simulink model "FullCardioLablModel"  (R2023b)
settings: Solver=FixedStepDiscrete  StartTime=0.0  StopTime=param_sim_time  FixedStep=1/fs  MaxStep=1/fs  RelTol=1e-3
undefined symbols (not defined in the file): analyses, fdesignblkfcn, fs, gcbh, param_tot_samples
libraries: dspstat3 x13, SCGAnalysis_SignalGenerationLib x2
(part 20 of 20)

== matlab function FullCardioLablModel/SCG Analysis/Enabled SCG Analysis Subsystem/All Signals Signal Metric Characterization/SCG Systolic 3DMinS1p2pProjection Signal Metric Characterization/Spectral Distribution Calculator/Spectral Distribution Calculator ==
  data: fs input size=[1]; r_pos input; scg_signal input; entire_cycle_nsd output size=[3 1]; entire_cycle_flag input size=[1]; s1_flag input size=[1]; s2_flag input size=[1]; f_band_lo input size=[1 2]; f_band_mid input size=[1 2]; f_band_hi input size=[1 2]; s1_nsd output size=[3 1]; s2_nsd output size=[3 1]
function [entire_cycle_nsd, s1_nsd, s2_nsd] = slk_normalized_spectral_distribution_calculator(fs, r_pos,scg_signal, entire_cycle_flag, s1_flag, s2_flag, f_band_lo, f_band_mid, f_band_hi)
% Simulink function to calculate the normalized spectral distribution of the power spectral densities of the entire cyle, the s1 complex, and the s2 complex, of an input SCG signal.

% INPUTS:
% fs = sampling frequency of scg_signal.
% r_pos = index positions of the R peaks of the ecg.
% scg_signal = signal to calculate its average cycle.
% entire_cycle_flag = flag to indicate the calculation of the entire cycle spectral distribution.
% s1_flag = flag to indicate the calculation of the S1 complex spectral distribution.
% s2_flag = flag to indicate the calculation of the S2 complex spectral distribution.

% OUTPUT:
% entire_cycle_nsd = normalized spectral distribution of the entire cycle (given as 3 elements corresponding to the spectral distribution in each of the 3 bins).
% s1_nsd = normalized spectral distribution of the s1 complex (given as 3 elements corresponding to the spectral distribution in each of the 3 bins).
% s2_nsd = normalized spectral distribution of the s2 complex (given as 3 elements corresponding to the spectral distribution in each of the 3 bins).

% This function consists of three parts:
% Part 1 - Calculation of the entire cycle normalized spectral distribution.
% Part 2 - Calculation of the S1 complex normalized spectral distribution.
% Part 3 - Calculation of the S2 complex normalized spectral distribution.

coder.extrinsic('legend');
coder.extrinsic('vline');

num_cycles = length(r_pos);

pad_size = 10*fs; % The length of the zero-padded vector used to obtain sufficient frequency resolution for the FFT.

PSDs = figure;
xlabel('Frequency (Hz)')
ylabel('Power Spectral Density (mg^2)')
xlim([0 f_band_hi(2)])
title('Power Spectral Densities')
hold on

freq_axis = fs*(0:pad_size/2)/pad_size; % Frequency axis for the FFT.

%% Part 1 - Calculation of the entire cycle normalized spectral distribution.


% if entire_cycle_flag
%     
%     current_cycle_padded = zeros(pad_size,1); % Pre-initializing for speed.
%     fft_entire_cycle_mag_2_sided = zeros(pad_size,1);
%     fft_entire_cycle_mag_1_sided = zeros(pad_size/2+1,num_cycles - 1);
%     
%     for i = 1:num_cycles - 1 % The last cycle isnt considered because it's not complete.
%         
%         current_cycle = scg_signal(r_pos(i):r_pos(i+1));
%         current_cycle_length = length(current_cycle); % In samples.
%         
%         % Ensuring the current cycle has an even number of samples - necessary for FFT calculation.
%         if mod(current_cycle_length,2) > 0
%             current_cycle_length = current_cycle_length - 1;
%             current_cycle(end) = [];
%         end
%                
%         current_cycle_padded = [current_cycle; zeros(pad_size - current_cycle_length,1)];
%         fft_entire_cycle = fft(current_cycle_padded); % (Complex) FFT values.
%         fft_entire_cycle_mag_2_sided = abs(fft_entire_cycle); % Two-sided Magnitude.
%         fft_entire_cycle_mag_1_sided(:,i) = fft_entire_cycle_mag_2_sided(1:length(current_cycle_padded)/2+1); % One-sided Magnitude.
%         fft_entire_cycle_mag_1_sided(2:end-1,i) = 2*fft_entire_cycle_mag_1_sided(2:end-1,i); % Multiplying by 2 to get total power (negative + positive frequencies).
%     end
%     
%     average_entire_cycle_fft = mean(fft_entire_cycle_mag_1_sided'); % The mean magnitude FFT spectrum.
%     
%     average_entire_cycle_psd = average_entire_cycle_fft.^2; % The power spectral density - the square of the magnitude spectrum.
%     
%     % Plotting.
%     figure(PSDs); hold on;
%     plot(freq_axis,average_entire_cycle_psd)
%     
%     % Integrating along the bands to get the bandpower.
%     entire_cycle_lo_power = trapz(ceil(f_band_lo(1)/freq_axis(2)):ceil(f_band_lo(2)/freq_axis(2)),average_entire_cycle_psd(ceil(f_band_lo(1)/freq_axis(2)):ceil(f_band_lo(2)/freq_axis(2))));
%     entire_cycle_mid_power = trapz(ceil(f_band_mid(1)/freq_axis(2)):ceil(f_band_mid(2)/freq_axis(2)),average_entire_cycle_psd(ceil(f_band_mid(1)/freq_axis(2)):ceil(f_band_mid(2)/freq_axis(2))));
%     entire_cycle_hi_power = trapz(ceil(f_band_hi(1)/freq_axis(2)):ceil(f_band_hi(2)/freq_axis(2)),average_entire_cycle_psd(ceil(f_band_hi(1)/freq_axis(2)):ceil(f_band_hi(2)/freq_axis(2))));
%     entire_cycle_total_power = trapz(ceil(f_band_lo(1)/freq_axis(2)):ceil(f_band_hi(2)/freq_axis(2)),average_entire_cycle_psd(ceil(f_band_lo(1)/freq_axis(2)):ceil(f_band_hi(2)/freq_axis(2))));
%     
%     % Dividing over total power to get the normalized spectral distribution (NSD).
%     normalized_entire_cycle_lo_power = entire_cycle_lo_power/entire_cycle_total_power;
%     normalized_entire_cycle_mid_power = entire_cycle_mid_power/entire_cycle_total_power;
%     normalized_entire_cycle_hi_power = entire_cycle_hi_power/entire_cycle_total_power;
%     
%     % Preparing outputs.
%     entire_cycle_nsd = [normalized_entire_cycle_lo_power;normalized_entire_cycle_mid_power;normalized_entire_cycle_hi_power];
%     
% else 
%     entire_cycle_nsd = [0; 0; 0];
% end


if entire_cycle_flag

    Interp_FFT_Cycle_Mag_1_Sided = zeros(num_cycles - 1, 10000); % Pre-initializing for speed.
    new_freq_axis_entire_cycle = linspace(0,fs/2,10000); % Interpolation frequency axis.

    for i = 1:num_cycles - 1 % The last cycle isnt considered because it's not complete.

        current_cycle = scg_signal(r_pos(i):r_pos(i+1));
        current_cycle_length = length(current_cycle); % In samples.

        % Ensuring the current cycle has an even number of samples - necessary for FFT calculation.
        if mod(current_cycle_length,2) > 0
            current_cycle_length = current_cycle_length - 1;
            current_cycle(end) = [];
        end

        FFT_Cycle = zeros(current_cycle_length,1); % Pre-initializing for speed.
        FFT_Cycle_Mag_2_Sided = zeros(current_cycle_length,1);
        FFT_Cycle_Mag_1_Sided = zeros(current_cycle_length/2+1,1);

        freq_axis_entire_cycle = fs*(0:current_cycle_length/2)/current_cycle_length; % Frequency axis for the FFT.

        % FFT of each individual cycle.
        FFT_Cycle = fft(current_cycle); % (Complex) FFT values.
        FFT_Cycle_Mag_2_Sided = abs(FFT_Cycle); % Two-sided Magnitude.
        FFT_Cycle_Mag_1_Sided = FFT_Cycle_Mag_2_Sided(1:current_cycle_length/2+1); % One-sided Magnitude.
        FFT_Cycle_Mag_1_Sided(2:end-1) = 2*FFT_Cycle_Mag_1_Sided(2:end-1); % Multiplying by 2 to get total power (negative + positive frequencies).

        % Interpolating to a new frequency axis. This is necessary because different cycles have different lenghts (and thus different FFT
        % lengths). To average the FFT across cycles, these must be interpolated to a particular fixed length.
        Interp_FFT_Cycle_Mag_1_Sided(i,:) = interp1(freq_axis_entire_cycle, FFT_Cycle_Mag_1_Sided, new_freq_axis_entire_cycle);

    end

    average_entire_cycle_FFT = mean(Interp_FFT_Cycle_Mag_1_Sided); % The mean magnitude FFT spectrum.

    average_entire_cycle_PSD = average_entire_cycle_FFT.^2; % The power spectral density - the square of the magnitude spectrum.

    % Plotting
    figure(PSDs);
    plot(new_freq_axis_entire_cycle,average_entire_cycle_PSD)

    % Integrating along the bands to get the bandpower.
    entire_cycle_lo_power = trapz(ceil(f_band_lo(1)/new_freq_axis_entire_cycle(2)):ceil(f_band_lo(2)/new_freq_axis_entire_cycle(2)),average_entire_cycle_PSD(ceil(f_band_lo(1)/new_freq_axis_entire_cycle(2)):ceil(f_band_lo(2)/new_freq_axis_entire_cycle(2))));
    entire_cycle_mid_power = trapz(ceil(f_band_mid(1)/new_freq_axis_entire_cycle(2)):ceil(f_band_mid(2)/new_freq_axis_entire_cycle(2)),average_entire_cycle_PSD(ceil(f_band_mid(1)/new_freq_axis_entire_cycle(2)):ceil(f_band_mid(2)/new_freq_axis_entire_cycle(2))));
    entire_cycle_hi_power = trapz(ceil(f_band_hi(1)/new_freq_axis_entire_cycle(2)):ceil(f_band_hi(2)/new_freq_axis_entire_cycle(2)),average_entire_cycle_PSD(ceil(f_band_hi(1)/new_freq_axis_entire_cycle(2)):ceil(f_band_hi(2)/new_freq_axis_entire_cycle(2))));
    entire_cycle_total_power = trapz(ceil(f_band_lo(1)/new_freq_axis_entire_cycle(2)):ceil(f_band_hi(2)/new_freq_axis_entire_cycle(2)),average_entire_cycle_PSD(ceil(f_band_lo(1)/new_freq_axis_entire_cycle(2)):ceil(f_band_hi(2)/new_freq_axis_entire_cycle(2))));

    % Dividing over total power to get the normalized spectral distribution (NSD).
    normalized_entire_cyce_lo_power = entire_cycle_lo_power/entire_cycle_total_power;
    normalized_entire_cyce_mid_power = entire_cycle_mid_power/entire_cycle_total_power;
    normalized_entire_cyce_hi_power = entire_cycle_hi_power/entire_cycle_total_power;

    % Preparing outputs.
    entire_cycle_nsd = [normalized_entire_cyce_lo_power;normalized_entire_cyce_mid_power;normalized_entire_cyce_hi_power];

    
else 
    entire_cycle_nsd = [0; 0; 0];

end

%% Part 2 - Calculation of the S1 complex normalized spectral distribution.

if s1_flag
    
    s1 = zeros(0.2*fs,1); % Pre-initializing for speed.
    s1_padded = zeros(pad_size,1);
    fft_s1_mag_2_sided = zeros(pad_size,1);
    fft_s1_mag_1_sided = zeros((pad_size)/2+1,num_cycles - 1);
    
    for i = 1:num_cycles - 1 % The last cycle isnt considered because there is a chance its S1 complex will be cut.
        s1 = scg_signal(r_pos(i):r_pos(i) + 0.2*fs - 1); % The S1 complex is considered as the 200ms following the ECG R peak.
        s1_padded = [s1; zeros(pad_size - 0.2*fs,1)];
        fft_s1 = fft(s1_padded); % (Complex) FFT values.
        fft_s1_mag_2_sided = abs(fft_s1); % Two-sided Magnitude.
        fft_s1_mag_1_sided(:,i) = fft_s1_mag_2_sided(1:length(s1_padded)/2+1); % One-sided Magnitude.
        fft_s1_mag_1_sided(2:end-1,i) = 2*fft_s1_mag_1_sided(2:end-1,i); % Multiplying by 2 to get total power (negative + positive frequencies).
    end
    
    average_s1_fft = mean(fft_s1_mag_1_sided'); % The mean magnitude FFT spectrum.
    
    average_s1_psd = average_s1_fft.^2; % The power spectral density - the square of the magnitude spectrum.
    
    % Plotting.
    figure(PSDs); hold on
    plot(freq_axis,average_s1_psd)
    
    % Integrating along the bands to get the bandpower.
    s1_lo_power = trapz(ceil(f_band_lo(1)/freq_axis(2)):ceil(f_band_lo(2)/freq_axis(2)),average_s1_psd(ceil(f_band_lo(1)/freq_axis(2)):ceil(f_band_lo(2)/freq_axis(2))));
    s1_mid_power = trapz(ceil(f_band_mid(1)/freq_axis(2)):ceil(f_band_mid(2)/freq_axis(2)),average_s1_psd(ceil(f_band_mid(1)/freq_axis(2)):ceil(f_band_mid(2)/freq_axis(2))));
    s1_hi_power = trapz(ceil(f_band_hi(1)/freq_axis(2)):ceil(f_band_hi(2)/freq_axis(2)),average_s1_psd(ceil(f_band_hi(1)/freq_axis(2)):ceil(f_band_hi(2)/freq_axis(2))));
    s1_total_power = trapz(ceil(f_band_lo(1)/freq_axis(2)):ceil(f_band_hi(2)/freq_axis(2)),average_s1_psd(ceil(f_band_lo(1)/freq_axis(2)):ceil(f_band_hi(2)/freq_axis(2))));
    
    % Dividing over total power to get the normalized spectral distribution (NSD).
    normalized_s1_lo_power = s1_lo_power/s1_total_power;
    normalized_s1_mid_power = s1_mid_power/s1_total_power;
    normalized_s1_hi_power = s1_hi_power/s1_total_power;
    
    % Preparing outputs.
    s1_nsd = [normalized_s1_lo_power;normalized_s1_mid_power;normalized_s1_hi_power];
    
else
    s1_nsd = [0; 0; 0;];
end

%% Part 3 - Calculation of the S2 complex normalized spectral distribution.

if s2_flag
    
    s2_search_window_lims = [0.25*fs 0.5*fs]; % The window initially used to search for the S2 peak within that cycle.
    s2_identify_window = 0.15*fs; % The window length centered about the S2 peak (in samples) used to identify the S2 complex.
    
    s2 = zeros(s2_identify_window,1); % Pre-initializing for speed.
    s2_padded = zeros(pad_size,1);
    fft_s2_mag_2_sided = zeros(pad_size,1);
    fft_s2_mag_1_sided = zeros((pad_size)/2+1,num_cycles - 1);
    
    for i = 1:num_cycles - 1 % The last cycle isnt considered because there is a chance its S1 complex will be cut.
        
        cycle = scg_signal(r_pos(i):r_pos(i+1)); % The current heart cycle.
        
        s2_search_window = cycle(s2_search_window_lims(1):s2_search_window_lims(2)); % Defining the window where to search for the S2 peak.
        s2peak = s2_search_window_lims(1) + find(abs(s2_search_window)==max(abs(s2_search_window))); % Identifying the S2 peak within 'cycle'.
        
        s2 = cycle(s2peak(1) - s2_identify_window/2 : s2peak(1) + s2_identify_window/2); % The S2 complex.
        s2_padded = [s2; zeros(pad_size - s2_identify_window - 1,1)]; % Padding the S2 complex with zeros.
        fft_s2 = fft(s2_padded); % (Complex) FFT values.
        fft_s2_mag_2_sided = abs(fft_s2); % Two-sided Magnitude.
        fft_s2_mag_1_sided(:,i) = fft_s2_mag_2_sided(1:length(s2_padded)/2+1); % One-sided Magnitude.
        fft_s2_mag_1_sided(2:end-1,i) = 2*fft_s2_mag_1_sided(2:end-1,i); % Multiplying by 2 to get total power (negative + positive frequencies).
    end
    
    average_s2_FFT = mean(fft_s2_mag_1_sided'); % The mean magnitude FFT spectrum.
    
    average_s2_PSD = average_s2_FFT.^2; % The power spectral density - the square of the magnitude spectrum.
    
    % Plotting.
    figure(PSDs); hold on;
    title('SCG 3D Systolic Min S1p2p Axis')
    plot(freq_axis,average_s2_PSD)
    
    % Integrating along the bands to get the bandpower.
    s2_lo_power = trapz(ceil(f_band_lo(1)/freq_axis(2)):ceil(f_band_lo(2)/freq_axis(2)),average_s2_PSD(ceil(f_band_lo(1)/freq_axis(2)):ceil(f_band_lo(2)/freq_axis(2))));
    s2_mid_power = trapz(ceil(f_band_mid(1)/freq_axis(2)):ceil(f_band_mid(2)/freq_axis(2)),average_s2_PSD(ceil(f_band_mid(1)/freq_axis(2)):ceil(f_band_mid(2)/freq_axis(2))));
    s2_hi_power = trapz(ceil(f_band_hi(1)/freq_axis(2)):ceil(f_band_hi(2)/freq_axis(2)),average_s2_PSD(ceil(f_band_hi(1)/freq_axis(2)):ceil(f_band_hi(2)/freq_axis(2))));
    s2_total_power = trapz(ceil(f_band_lo(1)/freq_axis(2)):ceil(f_band_hi(2)/freq_axis(2)),average_s2_PSD(ceil(f_band_lo(1)/freq_axis(2)):ceil(f_band_hi(2)/freq_axis(2))));
    
    % Dividing over total power to get the normalized spectral distribution (NSD).
    normalized_s2_lo_power = s2_lo_power/s2_total_power;
    normalized_s2_mid_power = s2_mid_power/s2_total_power;
    normalized_s2_hi_power = s2_hi_power/s2_total_power;
    
    % Preparing outputs.
    s2_nsd = [normalized_s2_lo_power;normalized_s2_mid_power;normalized_s2_hi_power];
    
else 
    s2_nsd = [0;0;0];    
end

% Plotting the frequency band delimiters
vline(f_band_lo(1),'r')
vline(f_band_mid(1),'r')
vline(f_band_hi(1),'r')
vline(f_band_hi(2),'r')

% Plotting the legend.
if entire_cycle_flag
    legend('Entire Cycle')
end

if s1_flag
    legend('S1')
end

if s2_flag
    legend('S2')
end

if entire_cycle_flag && s1_flag
    legend('Entire Cycle','S1')
end

if entire_cycle_flag && s2_flag
    legend('Entire Cycle','S2')
end

if s1_flag && s2_flag
    legend('S1','S2')
end

if entire_cycle_flag && s1_flag && s2_flag
    legend('Entire Cycle','S1','S2')
end

end

== matlab function FullCardioLablModel/SCG Analysis/Enabled SCG Analysis Subsystem/Systolic Interval Identification/Systolic Fiducial Point Marker/Preliminary Systolic Fiducial Point Identifier ==
  data: fs input size=[1]; MC_prelim output size=[4*ceil(param_sim_time) 1]; ecg_r_pos input; scg_s1_ref_signal input; IM_prelim output size=[4*ceil(param_sim_time) 1]; AO_prelim output size=[4*ceil(param_sim_time) 1]
function [MC_prelim, IM_prelim, AO_prelim] = slk_preliminary_systolic_fiducial_point_identifier(fs,ecg_r_pos, scg_s1_ref_signal)
% Function to identify the (preliminary) systolic hemodynamic fiducial points of the seismocardiogram (SCG) using an S1 reference signal.

% INPUTS:
% fs - the sampling frequency (in Hz).
% ecg_r_pos - the ECG R peaks.
% scg_s1_ref_signal - the SCG systolic reference signal used to perform a preliminary identificaiton of the SCG systolic fiducial points (ie. MC, IM, and AO).

% OUTPUTS:
% prelim_MC - preliminary sample indexes of mitral closure. 
% prelim_IM - preliminary sample indexes isovolumic moment.
% prelim_AO - preliminary sample indexes of aortic opening.

coder.extrinsic('legend')

IM_search_window_lim = [fs*0.02 fs*0.08]; % The search window limits for IM, in samples, defined in 'cycle'.
AO_search_window_size = fs*0.05; % The search window size, in samples, for AO. This search window is opened after IM and is open for the specified duration.

num_cycles = size(ecg_r_pos,1);

IM_prelim = zeros(num_cycles - 1 , 1);   % Pre-initalization for speed.
MC_prelim = zeros(num_cycles - 1 , 1);
AO_prelim = zeros(num_cycles - 1 , 1);

for i = 1:num_cycles - 1% The last cycle isn't considered because there's a good chance its SCG fiducial markers are cut off.
    
    cycle = scg_s1_ref_signal(ecg_r_pos(i):ecg_r_pos(i+1));
    
    %% Preliminary identifications based on the reference SCG signal. These fiducial markers follow the definition by Sorensen et. al 2018 (more or less)
    
    % IM - First, the isovolumic moment is detecetd (it is usually the most obvious marker) and then used to detect MC and AO.
    IM_prelim_search_window = cycle(IM_search_window_lim(1): IM_search_window_lim(2));
    IM_prelim_candies = find([islocalmin(IM_prelim_search_window)]); % IM_prelim candidates.
    IM_prelim_min_candy = IM_prelim_candies(find(IM_prelim_search_window(IM_prelim_candies) == min(IM_prelim_search_window(IM_prelim_candies)))); % IM_prelim is considered as the candidate with the most negative amplitude.  
    IM_prelim(i) = -2 + ecg_r_pos(i) + IM_search_window_lim(1) + IM_prelim_min_candy; % Defined as the sample position in scg_s1_ref_signal. The -2 is there to adjust for the 1-based indexing (two windows were considered).
   
    IM_prelim_candies = []; % Clearing.
    IM_prelim_min_candy = [];
    
    % MC.
    MC_prelim_search_window = scg_s1_ref_signal(ecg_r_pos(i):IM_prelim(i)) ; % Look for MC_prelim between the R wave peak and the detected IM_prelim
    MC_prelim_candies = find([islocalmax(MC_prelim_search_window)]); % MC_prelim candidates.
    if MC_prelim_candies % If local maxima have been detected, identify which is the greatest.
        MC_prelim_max_candy = MC_prelim_candies(find( MC_prelim_search_window(MC_prelim_candies) == max(MC_prelim_search_window(MC_prelim_candies)))); % MC_prelim is considered as the candidate with the largest amplitude. 
        MC_prelim(i) = -1 + ecg_r_pos(i) + MC_prelim_max_candy; % Defined as the sample position in scg_s1_ref_signal. The -1 is there to adjust for the 1-based indexing.
    end
    
    MC_prelim_candies = []; % Clearing
    MC_prelim_max_candy = [];
   
    %AO.
    AO_prelim_search_window = scg_s1_ref_signal(IM_prelim(i):IM_prelim(i) + AO_search_window_size);
    AO_prelim_candies = find([islocalmax(AO_prelim_search_window)]); % AO_prelim candidates.
    AO_prelim_min_candy = AO_prelim_candies(1);
    AO_prelim(i) = -1 + IM_prelim(i) + AO_prelim_min_candy; % Select the FIRST peak. The -1 is there to adjust for the 1-based indexing.
    
    AO_prelim_candies = []; % Clearing
    AO_prelim_max_candy = []; 
    
end


% Plotting
t = 0:1/fs:(length(scg_s1_ref_signal)-1)/fs;

figure; 
plot(t,scg_s1_ref_signal); hold on;
plot((IM_prelim-1)/fs, scg_s1_ref_signal(IM_prelim),'ro')
plot((MC_prelim-1)/fs, scg_s1_ref_signal(MC_prelim),'go')
plot((AO_prelim-1)/fs, scg_s1_ref_signal(AO_prelim),'bo')
box off

legend('SCG S1 Ref Signal', 'IM_P_r_e_l_i_m', 'MC_P_r_e_l_i_m', 'AO_P_r_e_l_i_m')

title('Preliminary Systolic Fiducial Markers')
xlabel('Time (sec)')
ylabel('Acceleration (mg)')

end

== matlab function FullCardioLablModel/SCG Analysis/Enabled SCG Analysis Subsystem/Signal Generation/3D Projections/MATLAB Function ==
  data: scg_xyz input; el_scg input size=[1]; projection output size=[param_tot_samples 1]; az_scg input size=[1]
function projection = slk_axis_projection(scg_xyz, el_scg, az_scg)

el_mat = el_scg;
az_mat = -1*az_scg;

[xhat_mat, yhat_mat, zhat_mat] = sph2cart(az_mat*pi/180,el_mat*pi/180,1);
% Converting to the SCG convention reference frame (this depends on the accelerometer and its placement orientation! - they should be such that they match the conventional SCG reference frame).
xhat_scg = xhat_mat;
yhat_scg = zhat_mat;
zhat_scg = -1*yhat_mat;

projection_axis = [xhat_scg yhat_scg zhat_scg];
    
projection = zeros(size(scg_xyz,1),1);
    
for i=1:size(scg_xyz,1)
    
    projection(i) = dot(scg_xyz(i,:),projection_axis);
    
end

figure;
ax = [0 0 0 0];

ax(1) = subplot(4,1,1); plot(scg_xyz(:,1),'b'); title('x'); box off; ylabel('Acceleration (mg)');
ax(2) = subplot(4,1,2); plot(scg_xyz(:,2),'b'); title('y'); box off; ylabel('Acceleration (mg)');
ax(3) = subplot(4,1,3); plot(scg_xyz(:,3),'b'); title('z'); box off; ylabel('Acceleration (mg)');
ax(4) = subplot(4,1,4); plot(projection,'g'); title('Systolic Mechanical Axis Projection'); box off; ylabel('Acceleration (mg)');
xlabel('Sample no.')
linkaxes(ax,'xy')
end

== matlab function FullCardioLablModel/SCG Analysis/Enabled SCG Analysis Subsystem/Signal Generation/3D Projections/MATLAB Function4 ==
  data: scg_xyz input; el_scg input size=[1]; projection output size=[param_tot_samples 1]; az_scg input size=[1]
function projection = slk_axis_projection(scg_xyz, el_scg, az_scg)

el_mat = el_scg;
az_mat = -1*az_scg;

[xhat_mat, yhat_mat, zhat_mat] = sph2cart(az_mat*pi/180,el_mat*pi/180,1);
% Converting to the SCG convention reference frame (this depends on the accelerometer and its placement orientation! - they should be such that they match the conventional SCG reference frame).
xhat_scg = xhat_mat;
yhat_scg = zhat_mat;
zhat_scg = -1*yhat_mat;

projection_axis = [xhat_scg yhat_scg zhat_scg];
    
projection = zeros(size(scg_xyz,1),1);
    
for i=1:size(scg_xyz,1)
    
    projection(i) = dot(scg_xyz(i,:),projection_axis);
    
end

figure;
ax = [0 0 0 0];

ax(1) = subplot(4,1,1); plot(scg_xyz(:,1),'b'); title('x'); box off; ylabel('Acceleration (mg)');
ax(2) = subplot(4,1,2); plot(scg_xyz(:,2),'b'); title('y'); box off; ylabel('Acceleration (mg)');
ax(3) = subplot(4,1,3); plot(scg_xyz(:,3),'b'); title('z'); box off; ylabel('Acceleration (mg)');
ax(4) = subplot(4,1,4); plot(projection,'g'); title('S2 Mechanical Axis Projection'); box off; ylabel('Acceleration (mg)');
xlabel('Sample no.')
linkaxes(ax,'xy')
end

== matlab function FullCardioLablModel/SCG Analysis/Enabled SCG Analysis Subsystem/Signal Generation/3D Projections/MATLAB Function5 ==
  data: scg_xyz input; el_scg input size=[1]; projection output size=[param_tot_samples 1]; az_scg input size=[1]
function projection = slk_axis_projection(scg_xyz, el_scg, az_scg)

el_mat = el_scg;
az_mat = -1*az_scg;

[xhat_mat, yhat_mat, zhat_mat] = sph2cart(az_mat*pi/180,el_mat*pi/180,1);
% Converting to the SCG convention reference frame (this depends on the accelerometer and its placement orientation! - they should be such that they match the conventional SCG reference frame).
xhat_scg = xhat_mat;
yhat_scg = zhat_mat;
zhat_scg = -1*yhat_mat;

projection_axis = [xhat_scg yhat_scg zhat_scg];
    
projection = zeros(size(scg_xyz,1),1);
    
for i=1:size(scg_xyz,1)
    
    projection(i) = dot(scg_xyz(i,:),projection_axis);
    
end

figure;
ax = [0 0 0 0];

ax(1) = subplot(4,1,1); plot(scg_xyz(:,1),'b'); title('x'); box off; ylabel('Acceleration (mg)');
ax(2) = subplot(4,1,2); plot(scg_xyz(:,2),'b'); title('y'); box off; ylabel('Acceleration (mg)');
ax(3) = subplot(4,1,3); plot(scg_xyz(:,3),'b'); title('z'); box off; ylabel('Acceleration (mg)');
ax(4) = subplot(4,1,4); plot(projection,'r'); title('S2 Antimechanical Axis Projection'); box off; ylabel('Acceleration (mg)');
xlabel('Sample no.')
linkaxes(ax,'xy')
end
